simulink model "Project_Papi_Rubber_Game_LQR_Sim"  (R2019a)
settings: Solver=FixedStepAuto  StartTime=0.0  StopTime=50  FixedStep=0.01  RelTol=1e-3
values from neighbouring files (symbols this model uses):
  A = [0 0 0 0 0 0 ... (first row only)    [Final_Code.m]
  B = [1 0 ... (first row only)    [Final_Code.m]
  C = [1 0 0 0 0 0 ... (first row only)    [Final_Code.m]
  ene = [ene4(1,1)+(dia3/2) ene4(1,2)+(dia3/2)]    [Final_Code.m]
  init_cond = [out.x_plant.Data(j,1); out.x_plant.Data(j,2); out.x_plant.Data(j,3); out.x_plant.Data(j,4); out.x_plant.Data(j,5); out.x_plant.Data(j,6)]    [Final_Code.m]
  K = [0 0 1 0 0 0 ... (first row only)    [Final_Code.m]
  K_lqr_sim = [K_lqr(1,3) 0; 0 K_lqr(2,4)]    [Final_Code.m]
  m = 1    [Final_Code.m]
  slop = [2 -1 3 -2]    [Final_Code.m]
libraries: simulink x2
settings Model: Creator=asjos  LastModifiedBy=asjos

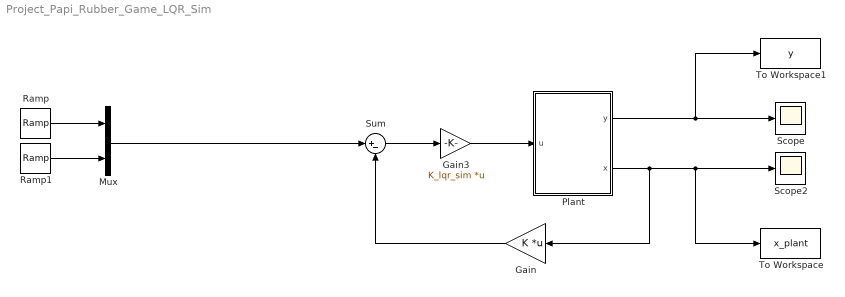
== system Project_Papi_Rubber_Game_LQR_Sim ==
  Gain : Gain  Gain=K  Multiplication=Matrix(K*u)
  Gain3 : Gain  Gain=K_lqr_sim  Multiplication=Matrix(K*u)
  Mux : Mux  Inputs=2
  Plant : Subsystem
  Ramp : simulink/Sources/Ramp  slope=slop(1,m)  start=0  InitialOutput=ene(1,1)
  Ramp1 : simulink/Sources/Ramp  slope=slop(1,m)  start=0  InitialOutput=ene(1,2)
  Scope : Scope
  Scope2 : Scope
  Sum : Sum  Inputs=|+-
  To Workspace : ToWorkspace  VariableName=x_plant  SaveFormat=Timeseries  SampleTime=-1
  To Workspace1 : ToWorkspace  VariableName=y  SaveFormat=Timeseries  SampleTime=-1
  wires:
  Plant/1(y) -> To Workspace1/1, Scope/1
  Sum/1 -> Gain3/1
  Gain/1 -> Sum/2
  Plant/2(x) -> Gain/1, To Workspace/1, Scope2/1
  Ramp/1 -> Mux/1
  Ramp1/1 -> Mux/2
  Gain3/1 -> Plant/1(u)
  Mux/1 -> Sum/1

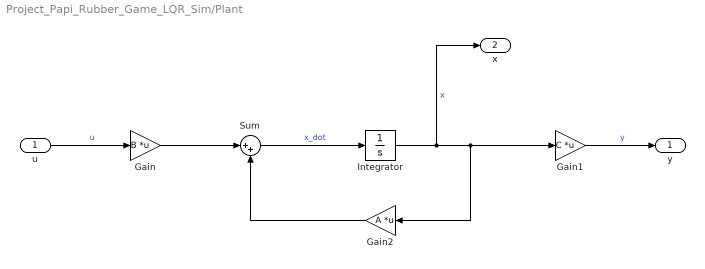
== system Project_Papi_Rubber_Game_LQR_Sim/Plant ==
  u : Inport
  Gain : Gain  Gain=B  Multiplication=Matrix(K*u)
  Gain1 : Gain  Gain=C  Multiplication=Matrix(K*u)
  Gain2 : Gain  Gain=A  Multiplication=Matrix(K*u)
  Integrator : Integrator  InitialCondition=init_cond
  Sum : Sum  Inputs=|++
  y : Outport
  x : Outport  Port=2
  wires:
  Integrator/1 -> x/1, Gain1/1, Gain2/1  "x"
  Gain2/1 -> Sum/2
  Gain/1 -> Sum/1
  Sum/1 -> Integrator/1  "x_dot"
  u/1 -> Gain/1  "u"
  Gain1/1 -> y/1  "y"
